simulink model "udp_send_receive"  (R2018a)
settings: Solver=FixedStepAuto  StartTime=0.0  StopTime=inf  FixedStep=1/200  RelTol=1e-3
libraries: instrumentlib x3, aerolibanimutils x1
settings Model: Creator=husibo  LastModifiedBy=husibo

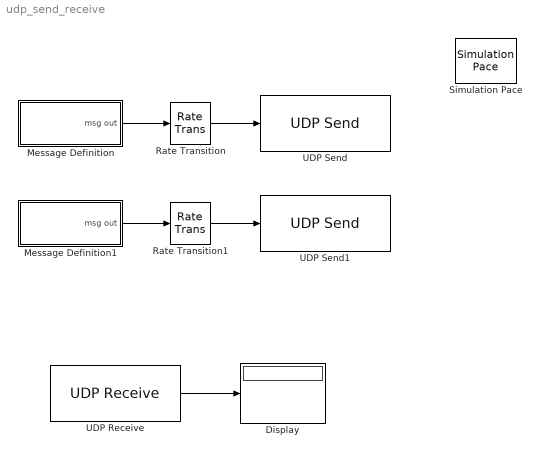
== system udp_send_receive ==
  Display : Display
  Message Definition : Subsystem
  Message Definition1 : Subsystem
  Rate Transition : RateTransition  OutPortSampleTime=0.01
  Rate Transition1 : RateTransition  OutPortSampleTime=0.01
  Simulation Pace : aerolibanimutils/Simulation Pace  SimulationPace=1  SleepMode=MATLAB Thread  OutputPaceError=off  SampleTime=1/200
  UDP Receive : instrumentlib/UDP Receive  Host=localhost  Port=3337  LocalPort=4337  EnablePortSharing=off  GetLatestData=off  DataSize=3  DataType=double  ASCIIFormatting=%f  Terminator=LF  ByteOrder=LittleEndian  EnableBlockingMode=on  Timeout=10  SampleTime=0.01  LocalAddress=127.0.0.1
      settings: SourceProductName=Instrument Control Toolbox
  UDP Send : instrumentlib/UDP Send  Host=127.0.0.1  Port=2337  LocalPort=1337  EnablePortSharing=off  ByteOrder=LittleEndian  OutputDatagramPacketSize=512  EnableBlockingMode=on  LocalAddress=0.0.0.0
      settings: SourceProductName=Instrument Control Toolbox
  UDP Send1 : instrumentlib/UDP Send  Host=127.0.0.1  Port=6337  LocalPort=5337  EnablePortSharing=off  ByteOrder=LittleEndian  OutputDatagramPacketSize=512  EnableBlockingMode=on  LocalAddress=0.0.0.0
      settings: SourceProductName=Instrument Control Toolbox
  wires:
  Message Definition/1(msg out) -> Rate Transition/1
  Rate Transition/1 -> UDP Send/1
  UDP Receive/1 -> Display/1
  Message Definition1/1(msg out) -> Rate Transition1/1
  Rate Transition1/1 -> UDP Send1/1

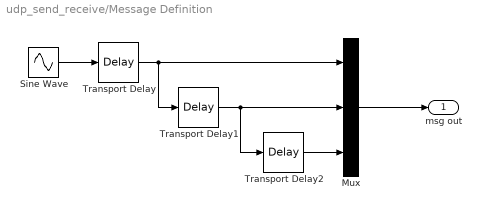
== system udp_send_receive/Message Definition ==
  Mux : Mux  Inputs=3
  Sine Wave : Sin  SampleTime=0
  Transport Delay : TransportDelay  DelayTime=2
  Transport Delay1 : TransportDelay  DelayTime=2
  Transport Delay2 : TransportDelay  DelayTime=2
  msg out : Outport
  wires:
  Sine Wave/1 -> Transport Delay/1
  Transport Delay/1 -> Mux/1, Transport Delay1/1
  Transport Delay1/1 -> Mux/2, Transport Delay2/1
  Transport Delay2/1 -> Mux/3
  Mux/1 -> msg out/1

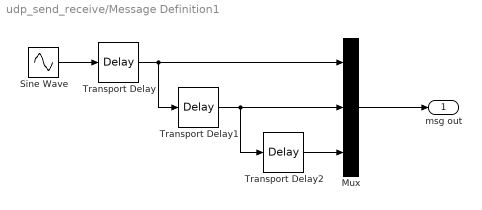
== system udp_send_receive/Message Definition1 ==
  Mux : Mux  Inputs=3
  Sine Wave : Sin  SampleTime=0
  Transport Delay : TransportDelay  DelayTime=2
  Transport Delay1 : TransportDelay  DelayTime=2
  Transport Delay2 : TransportDelay  DelayTime=2
  msg out : Outport
  wires:
  Sine Wave/1 -> Transport Delay/1
  Transport Delay/1 -> Mux/1, Transport Delay1/1
  Transport Delay1/1 -> Mux/2, Transport Delay2/1
  Transport Delay2/1 -> Mux/3
  Mux/1 -> msg out/1
